simulink library "Lib_SimpleCopter"  (R2014b)
settings: Solver=ode45  StartTime=0.0  StopTime=10.0  RelTol=1e-3
settings Model: Creator=Ehang  LastModifiedBy=Ehang

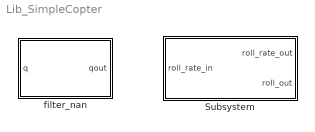
== system Lib_SimpleCopter ==
  Subsystem : Subsystem
  filter_nan : MATLAB Function  TreatAsAtomicUnit=on

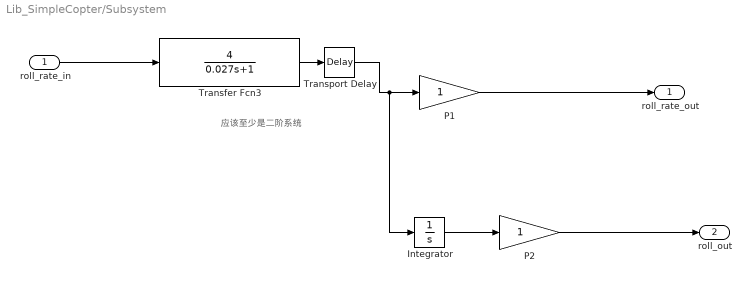
== system Lib_SimpleCopter/Subsystem ==
  note: 应该至少是二阶系统
  roll_rate_in : Inport
  Integrator : Integrator
  P1 : Gain
  P2 : Gain
  Transfer Fcn3 : TransferFcn  Numerator=[4]  Denominator=[0.027 1]  AbsoluteTolerance=1e-19
  Transport Delay : TransportDelay  DelayTime=0.02606
  roll_rate_out : Outport
  roll_out : Outport  Port=2
  wires:
  roll_rate_in/1 -> Transfer Fcn3/1
  Integrator/1 -> P2/1
  Transfer Fcn3/1 -> Transport Delay/1
  P2/1 -> roll_out/1
  P1/1 -> roll_rate_out/1
  Transport Delay/1 -> P1/1, Integrator/1

== matlab function Lib_SimpleCopter/filter_nan ==
  data: q input; qout output
function qout=filter_nan(q)
%#codegen
if isnan(q)
qout=0;
else
    qout=q;
end
